simulink model "EarlyReturn18_2018a"  (R2018a)
settings: Solver=VariableStepAuto  StartTime=0.0  StopTime=0.1  RelTol=1e-3
settings Model: Creator=BEAR  LastModifiedBy=bzhan

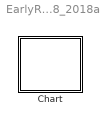
== system EarlyReturn18_2018a ==
  Chart : Stateflow chart  TreatAsAtomicUnit=on

== stateflow chart EarlyReturn18_2018a/Chart ==
  settings: updateMethod=DISCRETE  sampleTime=0.1
  state S
    en: f("enS")
    du: f("duS")
    ex: f("exS")
    (junction 15) -> S : {E;f("ca2")}
    S -> (junction 15) [order 1] : {f("ca1")}
  state T
    en: f("enT")
  (default) -> S
  S -> T [order 1] : E
  data: s function_input
  events: E local FUNCTION_CALL_EVENT
  function f(s):
    | function f(s)
    |   fprintf(s+"\n");
